simulink model "gm_MATE_HDLsolver_myFirstCircuit"  (R2024b)
settings: Solver=FixedStepDiscrete  StartTime=0.0  StopTime=0.05  FixedStep=6.02409638554217e-09  MaxStep=100e-6  RelTol=1e-4
PostLoadFcn:
  | Ts=1e-6; nb_sw=3; nb_lc=2;nb_r=1;nb_src=1; nb_out=3; rL=1.2;rC=100;L=1e-3; C=1e-5; LpejoSw=1e-6;h=Ts; MAX_INPUTS=16;
  | MAX_OUTPUTS=16;
  | MAX_SWITCHES=8;
  | MAX_INPUTS=16;
InitFcn:
  | Ts=1e-6; nb_sw=3; nb_lc=2;nb_r=1;nb_src=1; nb_out=3; rL=1.2;rC=100;L=1e-3; C=1e-5; LpejoSw=1e-6;h=Ts; MAX_INPUTS=16;
  | MAX_OUTPUTS=16;
  | MAX_SWITCHES=8;
  | MAX_INPUTS=16;
undefined symbols (not defined in the file or in its folder): MATE_SOC
libraries: fl_lib x31, nesl_utility x13, hdlmdlgenlib x10, simetranss x5, simulink x4, hdlsllib x3, ee_lib x2, eeGeneralControl x1
(part 7 of 8)

== system gm_MATE_HDLsolver_myFirstCircuit/ForFPGA/mul_Dot Product5_dotp_11 ==
  In1 : Inport
  In2 : Inport  Port=2
  mul_Dot Product5_dotp_11 : Product  Inputs=**  OutDataTypeStr=single  SampleTime=6.02409638554217e-09
  mul_Dot Product5_dotp_11_pd1 : Delay  DelayLength=6
  Out1 : Outport
  wires:
  In1/1 -> mul_Dot Product5_dotp_11/1
  In2/1 -> mul_Dot Product5_dotp_11/2
  mul_Dot Product5_dotp_11/1 -> mul_Dot Product5_dotp_11_pd1/1
  mul_Dot Product5_dotp_11_pd1/1 -> Out1/1

== system gm_MATE_HDLsolver_myFirstCircuit/ForFPGA/mul_Dot Product5_dotp_12 ==
  In1 : Inport
  In2 : Inport  Port=2
  mul_Dot Product5_dotp_12 : Product  Inputs=**  OutDataTypeStr=single  SampleTime=6.02409638554217e-09
  mul_Dot Product5_dotp_12_pd1 : Delay  DelayLength=6
  Out1 : Outport
  wires:
  In1/1 -> mul_Dot Product5_dotp_12/1
  In2/1 -> mul_Dot Product5_dotp_12/2
  mul_Dot Product5_dotp_12/1 -> mul_Dot Product5_dotp_12_pd1/1
  mul_Dot Product5_dotp_12_pd1/1 -> Out1/1

== system gm_MATE_HDLsolver_myFirstCircuit/ForFPGA/mul_Dot Product5_dotp_13 ==
  In1 : Inport
  In2 : Inport  Port=2
  mul_Dot Product5_dotp_13 : Product  Inputs=**  OutDataTypeStr=single  SampleTime=6.02409638554217e-09
  mul_Dot Product5_dotp_13_pd1 : Delay  DelayLength=6
  Out1 : Outport
  wires:
  In1/1 -> mul_Dot Product5_dotp_13/1
  In2/1 -> mul_Dot Product5_dotp_13/2
  mul_Dot Product5_dotp_13/1 -> mul_Dot Product5_dotp_13_pd1/1
  mul_Dot Product5_dotp_13_pd1/1 -> Out1/1

== system gm_MATE_HDLsolver_myFirstCircuit/ForFPGA/mul_Dot Product5_dotp_14 ==
  In1 : Inport
  In2 : Inport  Port=2
  mul_Dot Product5_dotp_14 : Product  Inputs=**  OutDataTypeStr=single  SampleTime=6.02409638554217e-09
  mul_Dot Product5_dotp_14_pd1 : Delay  DelayLength=6
  Out1 : Outport
  wires:
  In1/1 -> mul_Dot Product5_dotp_14/1
  In2/1 -> mul_Dot Product5_dotp_14/2
  mul_Dot Product5_dotp_14/1 -> mul_Dot Product5_dotp_14_pd1/1
  mul_Dot Product5_dotp_14_pd1/1 -> Out1/1

== system gm_MATE_HDLsolver_myFirstCircuit/ForFPGA/mul_Dot Product5_dotp_15 ==
  In1 : Inport
  In2 : Inport  Port=2
  mul_Dot Product5_dotp_15 : Product  Inputs=**  OutDataTypeStr=single  SampleTime=6.02409638554217e-09
  mul_Dot Product5_dotp_15_pd1 : Delay  DelayLength=6
  Out1 : Outport
  wires:
  In1/1 -> mul_Dot Product5_dotp_15/1
  In2/1 -> mul_Dot Product5_dotp_15/2
  mul_Dot Product5_dotp_15/1 -> mul_Dot Product5_dotp_15_pd1/1
  mul_Dot Product5_dotp_15_pd1/1 -> Out1/1

== system gm_MATE_HDLsolver_myFirstCircuit/ForFPGA/mul_Dot Product5_dotp_2 ==
  In1 : Inport
  In2 : Inport  Port=2
  mul_Dot Product5_dotp_2 : Product  Inputs=**  OutDataTypeStr=single  SampleTime=6.02409638554217e-09
  mul_Dot Product5_dotp_2_pd1 : Delay  DelayLength=6
  Out1 : Outport
  wires:
  In1/1 -> mul_Dot Product5_dotp_2/1
  In2/1 -> mul_Dot Product5_dotp_2/2
  mul_Dot Product5_dotp_2/1 -> mul_Dot Product5_dotp_2_pd1/1
  mul_Dot Product5_dotp_2_pd1/1 -> Out1/1

== system gm_MATE_HDLsolver_myFirstCircuit/ForFPGA/mul_Dot Product5_dotp_3 ==
  In1 : Inport
  In2 : Inport  Port=2
  mul_Dot Product5_dotp_3 : Product  Inputs=**  OutDataTypeStr=single  SampleTime=6.02409638554217e-09
  mul_Dot Product5_dotp_3_pd1 : Delay  DelayLength=6
  Out1 : Outport
  wires:
  In1/1 -> mul_Dot Product5_dotp_3/1
  In2/1 -> mul_Dot Product5_dotp_3/2
  mul_Dot Product5_dotp_3/1 -> mul_Dot Product5_dotp_3_pd1/1
  mul_Dot Product5_dotp_3_pd1/1 -> Out1/1

== system gm_MATE_HDLsolver_myFirstCircuit/ForFPGA/mul_Dot Product5_dotp_4 ==
  In1 : Inport
  In2 : Inport  Port=2
  mul_Dot Product5_dotp_4 : Product  Inputs=**  OutDataTypeStr=single  SampleTime=6.02409638554217e-09
  mul_Dot Product5_dotp_4_pd1 : Delay  DelayLength=6
  Out1 : Outport
  wires:
  In1/1 -> mul_Dot Product5_dotp_4/1
  In2/1 -> mul_Dot Product5_dotp_4/2
  mul_Dot Product5_dotp_4/1 -> mul_Dot Product5_dotp_4_pd1/1
  mul_Dot Product5_dotp_4_pd1/1 -> Out1/1

== system gm_MATE_HDLsolver_myFirstCircuit/ForFPGA/mul_Dot Product5_dotp_5 ==
  In1 : Inport
  In2 : Inport  Port=2
  mul_Dot Product5_dotp_5 : Product  Inputs=**  OutDataTypeStr=single  SampleTime=6.02409638554217e-09
  mul_Dot Product5_dotp_5_pd1 : Delay  DelayLength=6
  Out1 : Outport
  wires:
  In1/1 -> mul_Dot Product5_dotp_5/1
  In2/1 -> mul_Dot Product5_dotp_5/2
  mul_Dot Product5_dotp_5/1 -> mul_Dot Product5_dotp_5_pd1/1
  mul_Dot Product5_dotp_5_pd1/1 -> Out1/1

== system gm_MATE_HDLsolver_myFirstCircuit/ForFPGA/mul_Dot Product5_dotp_6 ==
  In1 : Inport
  In2 : Inport  Port=2
  mul_Dot Product5_dotp_6 : Product  Inputs=**  OutDataTypeStr=single  SampleTime=6.02409638554217e-09
  mul_Dot Product5_dotp_6_pd1 : Delay  DelayLength=6
  Out1 : Outport
  wires:
  In1/1 -> mul_Dot Product5_dotp_6/1
  In2/1 -> mul_Dot Product5_dotp_6/2
  mul_Dot Product5_dotp_6/1 -> mul_Dot Product5_dotp_6_pd1/1
  mul_Dot Product5_dotp_6_pd1/1 -> Out1/1

== system gm_MATE_HDLsolver_myFirstCircuit/ForFPGA/mul_Dot Product5_dotp_7 ==
  In1 : Inport
  In2 : Inport  Port=2
  mul_Dot Product5_dotp_7 : Product  Inputs=**  OutDataTypeStr=single  SampleTime=6.02409638554217e-09
  mul_Dot Product5_dotp_7_pd1 : Delay  DelayLength=6
  Out1 : Outport
  wires:
  In1/1 -> mul_Dot Product5_dotp_7/1
  In2/1 -> mul_Dot Product5_dotp_7/2
  mul_Dot Product5_dotp_7/1 -> mul_Dot Product5_dotp_7_pd1/1
  mul_Dot Product5_dotp_7_pd1/1 -> Out1/1

== system gm_MATE_HDLsolver_myFirstCircuit/ForFPGA/mul_Dot Product5_dotp_8 ==
  In1 : Inport
  In2 : Inport  Port=2
  mul_Dot Product5_dotp_8 : Product  Inputs=**  OutDataTypeStr=single  SampleTime=6.02409638554217e-09
  mul_Dot Product5_dotp_8_pd1 : Delay  DelayLength=6
  Out1 : Outport
  wires:
  In1/1 -> mul_Dot Product5_dotp_8/1
  In2/1 -> mul_Dot Product5_dotp_8/2
  mul_Dot Product5_dotp_8/1 -> mul_Dot Product5_dotp_8_pd1/1
  mul_Dot Product5_dotp_8_pd1/1 -> Out1/1

== system gm_MATE_HDLsolver_myFirstCircuit/ForFPGA/mul_Dot Product5_dotp_9 ==
  In1 : Inport
  In2 : Inport  Port=2
  mul_Dot Product5_dotp_9 : Product  Inputs=**  OutDataTypeStr=single  SampleTime=6.02409638554217e-09
  mul_Dot Product5_dotp_9_pd1 : Delay  DelayLength=6
  Out1 : Outport
  wires:
  In1/1 -> mul_Dot Product5_dotp_9/1
  In2/1 -> mul_Dot Product5_dotp_9/2
  mul_Dot Product5_dotp_9/1 -> mul_Dot Product5_dotp_9_pd1/1
  mul_Dot Product5_dotp_9_pd1/1 -> Out1/1

== system gm_MATE_HDLsolver_myFirstCircuit/ForFPGA/mul_Dot Product6_dotp_0 ==
  In1 : Inport
  In2 : Inport  Port=2
  mul_Dot Product6_dotp_0 : Product  Inputs=**  OutDataTypeStr=single  SampleTime=6.02409638554217e-09
  mul_Dot Product6_dotp_0_pd1 : Delay  DelayLength=6
  Out1 : Outport
  wires:
  In1/1 -> mul_Dot Product6_dotp_0/1
  In2/1 -> mul_Dot Product6_dotp_0/2
  mul_Dot Product6_dotp_0/1 -> mul_Dot Product6_dotp_0_pd1/1
  mul_Dot Product6_dotp_0_pd1/1 -> Out1/1

== system gm_MATE_HDLsolver_myFirstCircuit/ForFPGA/mul_Dot Product6_dotp_1 ==
  In1 : Inport
  In2 : Inport  Port=2
  mul_Dot Product6_dotp_1 : Product  Inputs=**  OutDataTypeStr=single  SampleTime=6.02409638554217e-09
  mul_Dot Product6_dotp_1_pd1 : Delay  DelayLength=6
  Out1 : Outport
  wires:
  In1/1 -> mul_Dot Product6_dotp_1/1
  In2/1 -> mul_Dot Product6_dotp_1/2
  mul_Dot Product6_dotp_1/1 -> mul_Dot Product6_dotp_1_pd1/1
  mul_Dot Product6_dotp_1_pd1/1 -> Out1/1

== system gm_MATE_HDLsolver_myFirstCircuit/ForFPGA/mul_Dot Product6_dotp_10 ==
  In1 : Inport
  In2 : Inport  Port=2
  mul_Dot Product6_dotp_10 : Product  Inputs=**  OutDataTypeStr=single  SampleTime=6.02409638554217e-09
  mul_Dot Product6_dotp_10_pd1 : Delay  DelayLength=6
  Out1 : Outport
  wires:
  In1/1 -> mul_Dot Product6_dotp_10/1
  In2/1 -> mul_Dot Product6_dotp_10/2
  mul_Dot Product6_dotp_10/1 -> mul_Dot Product6_dotp_10_pd1/1
  mul_Dot Product6_dotp_10_pd1/1 -> Out1/1

== system gm_MATE_HDLsolver_myFirstCircuit/ForFPGA/mul_Dot Product6_dotp_11 ==
  In1 : Inport
  In2 : Inport  Port=2
  mul_Dot Product6_dotp_11 : Product  Inputs=**  OutDataTypeStr=single  SampleTime=6.02409638554217e-09
  mul_Dot Product6_dotp_11_pd1 : Delay  DelayLength=6
  Out1 : Outport
  wires:
  In1/1 -> mul_Dot Product6_dotp_11/1
  In2/1 -> mul_Dot Product6_dotp_11/2
  mul_Dot Product6_dotp_11/1 -> mul_Dot Product6_dotp_11_pd1/1
  mul_Dot Product6_dotp_11_pd1/1 -> Out1/1

== system gm_MATE_HDLsolver_myFirstCircuit/ForFPGA/mul_Dot Product6_dotp_12 ==
  In1 : Inport
  In2 : Inport  Port=2
  mul_Dot Product6_dotp_12 : Product  Inputs=**  OutDataTypeStr=single  SampleTime=6.02409638554217e-09
  mul_Dot Product6_dotp_12_pd1 : Delay  DelayLength=6
  Out1 : Outport
  wires:
  In1/1 -> mul_Dot Product6_dotp_12/1
  In2/1 -> mul_Dot Product6_dotp_12/2
  mul_Dot Product6_dotp_12/1 -> mul_Dot Product6_dotp_12_pd1/1
  mul_Dot Product6_dotp_12_pd1/1 -> Out1/1

== system gm_MATE_HDLsolver_myFirstCircuit/ForFPGA/mul_Dot Product6_dotp_13 ==
  In1 : Inport
  In2 : Inport  Port=2
  mul_Dot Product6_dotp_13 : Product  Inputs=**  OutDataTypeStr=single  SampleTime=6.02409638554217e-09
  mul_Dot Product6_dotp_13_pd1 : Delay  DelayLength=6
  Out1 : Outport
  wires:
  In1/1 -> mul_Dot Product6_dotp_13/1
  In2/1 -> mul_Dot Product6_dotp_13/2
  mul_Dot Product6_dotp_13/1 -> mul_Dot Product6_dotp_13_pd1/1
  mul_Dot Product6_dotp_13_pd1/1 -> Out1/1

== system gm_MATE_HDLsolver_myFirstCircuit/ForFPGA/mul_Dot Product6_dotp_14 ==
  In1 : Inport
  In2 : Inport  Port=2
  mul_Dot Product6_dotp_14 : Product  Inputs=**  OutDataTypeStr=single  SampleTime=6.02409638554217e-09
  mul_Dot Product6_dotp_14_pd1 : Delay  DelayLength=6
  Out1 : Outport
  wires:
  In1/1 -> mul_Dot Product6_dotp_14/1
  In2/1 -> mul_Dot Product6_dotp_14/2
  mul_Dot Product6_dotp_14/1 -> mul_Dot Product6_dotp_14_pd1/1
  mul_Dot Product6_dotp_14_pd1/1 -> Out1/1

== system gm_MATE_HDLsolver_myFirstCircuit/ForFPGA/mul_Dot Product6_dotp_15 ==
  In1 : Inport
  In2 : Inport  Port=2
  mul_Dot Product6_dotp_15 : Product  Inputs=**  OutDataTypeStr=single  SampleTime=6.02409638554217e-09
  mul_Dot Product6_dotp_15_pd1 : Delay  DelayLength=6
  Out1 : Outport
  wires:
  In1/1 -> mul_Dot Product6_dotp_15/1
  In2/1 -> mul_Dot Product6_dotp_15/2
  mul_Dot Product6_dotp_15/1 -> mul_Dot Product6_dotp_15_pd1/1
  mul_Dot Product6_dotp_15_pd1/1 -> Out1/1

== system gm_MATE_HDLsolver_myFirstCircuit/ForFPGA/mul_Dot Product6_dotp_2 ==
  In1 : Inport
  In2 : Inport  Port=2
  mul_Dot Product6_dotp_2 : Product  Inputs=**  OutDataTypeStr=single  SampleTime=6.02409638554217e-09
  mul_Dot Product6_dotp_2_pd1 : Delay  DelayLength=6
  Out1 : Outport
  wires:
  In1/1 -> mul_Dot Product6_dotp_2/1
  In2/1 -> mul_Dot Product6_dotp_2/2
  mul_Dot Product6_dotp_2/1 -> mul_Dot Product6_dotp_2_pd1/1
  mul_Dot Product6_dotp_2_pd1/1 -> Out1/1

== system gm_MATE_HDLsolver_myFirstCircuit/ForFPGA/mul_Dot Product6_dotp_3 ==
  In1 : Inport
  In2 : Inport  Port=2
  mul_Dot Product6_dotp_3 : Product  Inputs=**  OutDataTypeStr=single  SampleTime=6.02409638554217e-09
  mul_Dot Product6_dotp_3_pd1 : Delay  DelayLength=6
  Out1 : Outport
  wires:
  In1/1 -> mul_Dot Product6_dotp_3/1
  In2/1 -> mul_Dot Product6_dotp_3/2
  mul_Dot Product6_dotp_3/1 -> mul_Dot Product6_dotp_3_pd1/1
  mul_Dot Product6_dotp_3_pd1/1 -> Out1/1

== system gm_MATE_HDLsolver_myFirstCircuit/ForFPGA/mul_Dot Product6_dotp_4 ==
  In1 : Inport
  In2 : Inport  Port=2
  mul_Dot Product6_dotp_4 : Product  Inputs=**  OutDataTypeStr=single  SampleTime=6.02409638554217e-09
  mul_Dot Product6_dotp_4_pd1 : Delay  DelayLength=6
  Out1 : Outport
  wires:
  In1/1 -> mul_Dot Product6_dotp_4/1
  In2/1 -> mul_Dot Product6_dotp_4/2
  mul_Dot Product6_dotp_4/1 -> mul_Dot Product6_dotp_4_pd1/1
  mul_Dot Product6_dotp_4_pd1/1 -> Out1/1

== system gm_MATE_HDLsolver_myFirstCircuit/ForFPGA/mul_Dot Product6_dotp_5 ==
  In1 : Inport
  In2 : Inport  Port=2
  mul_Dot Product6_dotp_5 : Product  Inputs=**  OutDataTypeStr=single  SampleTime=6.02409638554217e-09
  mul_Dot Product6_dotp_5_pd1 : Delay  DelayLength=6
  Out1 : Outport
  wires:
  In1/1 -> mul_Dot Product6_dotp_5/1
  In2/1 -> mul_Dot Product6_dotp_5/2
  mul_Dot Product6_dotp_5/1 -> mul_Dot Product6_dotp_5_pd1/1
  mul_Dot Product6_dotp_5_pd1/1 -> Out1/1

== system gm_MATE_HDLsolver_myFirstCircuit/ForFPGA/mul_Dot Product6_dotp_6 ==
  In1 : Inport
  In2 : Inport  Port=2
  mul_Dot Product6_dotp_6 : Product  Inputs=**  OutDataTypeStr=single  SampleTime=6.02409638554217e-09
  mul_Dot Product6_dotp_6_pd1 : Delay  DelayLength=6
  Out1 : Outport
  wires:
  In1/1 -> mul_Dot Product6_dotp_6/1
  In2/1 -> mul_Dot Product6_dotp_6/2
  mul_Dot Product6_dotp_6/1 -> mul_Dot Product6_dotp_6_pd1/1
  mul_Dot Product6_dotp_6_pd1/1 -> Out1/1

== system gm_MATE_HDLsolver_myFirstCircuit/ForFPGA/mul_Dot Product6_dotp_7 ==
  In1 : Inport
  In2 : Inport  Port=2
  mul_Dot Product6_dotp_7 : Product  Inputs=**  OutDataTypeStr=single  SampleTime=6.02409638554217e-09
  mul_Dot Product6_dotp_7_pd1 : Delay  DelayLength=6
  Out1 : Outport
  wires:
  In1/1 -> mul_Dot Product6_dotp_7/1
  In2/1 -> mul_Dot Product6_dotp_7/2
  mul_Dot Product6_dotp_7/1 -> mul_Dot Product6_dotp_7_pd1/1
  mul_Dot Product6_dotp_7_pd1/1 -> Out1/1

== system gm_MATE_HDLsolver_myFirstCircuit/ForFPGA/mul_Dot Product6_dotp_8 ==
  In1 : Inport
  In2 : Inport  Port=2
  mul_Dot Product6_dotp_8 : Product  Inputs=**  OutDataTypeStr=single  SampleTime=6.02409638554217e-09
  mul_Dot Product6_dotp_8_pd1 : Delay  DelayLength=6
  Out1 : Outport
  wires:
  In1/1 -> mul_Dot Product6_dotp_8/1
  In2/1 -> mul_Dot Product6_dotp_8/2
  mul_Dot Product6_dotp_8/1 -> mul_Dot Product6_dotp_8_pd1/1
  mul_Dot Product6_dotp_8_pd1/1 -> Out1/1

== system gm_MATE_HDLsolver_myFirstCircuit/ForFPGA/mul_Dot Product6_dotp_9 ==
  In1 : Inport
  In2 : Inport  Port=2
  mul_Dot Product6_dotp_9 : Product  Inputs=**  OutDataTypeStr=single  SampleTime=6.02409638554217e-09
  mul_Dot Product6_dotp_9_pd1 : Delay  DelayLength=6
  Out1 : Outport
  wires:
  In1/1 -> mul_Dot Product6_dotp_9/1
  In2/1 -> mul_Dot Product6_dotp_9/2
  mul_Dot Product6_dotp_9/1 -> mul_Dot Product6_dotp_9_pd1/1
  mul_Dot Product6_dotp_9_pd1/1 -> Out1/1

== system gm_MATE_HDLsolver_myFirstCircuit/ForFPGA/mul_Dot Product7_dotp_0 ==
  In1 : Inport
  In2 : Inport  Port=2
  mul_Dot Product7_dotp_0 : Product  Inputs=**  OutDataTypeStr=single  SampleTime=6.02409638554217e-09
  mul_Dot Product7_dotp_0_pd1 : Delay  DelayLength=6
  Out1 : Outport
  wires:
  In1/1 -> mul_Dot Product7_dotp_0/1
  In2/1 -> mul_Dot Product7_dotp_0/2
  mul_Dot Product7_dotp_0/1 -> mul_Dot Product7_dotp_0_pd1/1
  mul_Dot Product7_dotp_0_pd1/1 -> Out1/1

== system gm_MATE_HDLsolver_myFirstCircuit/ForFPGA/mul_Dot Product7_dotp_1 ==
  In1 : Inport
  In2 : Inport  Port=2
  mul_Dot Product7_dotp_1 : Product  Inputs=**  OutDataTypeStr=single  SampleTime=6.02409638554217e-09
  mul_Dot Product7_dotp_1_pd1 : Delay  DelayLength=6
  Out1 : Outport
  wires:
  In1/1 -> mul_Dot Product7_dotp_1/1
  In2/1 -> mul_Dot Product7_dotp_1/2
  mul_Dot Product7_dotp_1/1 -> mul_Dot Product7_dotp_1_pd1/1
  mul_Dot Product7_dotp_1_pd1/1 -> Out1/1

== system gm_MATE_HDLsolver_myFirstCircuit/ForFPGA/mul_Dot Product7_dotp_10 ==
  In1 : Inport
  In2 : Inport  Port=2
  mul_Dot Product7_dotp_10 : Product  Inputs=**  OutDataTypeStr=single  SampleTime=6.02409638554217e-09
  mul_Dot Product7_dotp_10_pd1 : Delay  DelayLength=6
  Out1 : Outport
  wires:
  In1/1 -> mul_Dot Product7_dotp_10/1
  In2/1 -> mul_Dot Product7_dotp_10/2
  mul_Dot Product7_dotp_10/1 -> mul_Dot Product7_dotp_10_pd1/1
  mul_Dot Product7_dotp_10_pd1/1 -> Out1/1

== system gm_MATE_HDLsolver_myFirstCircuit/ForFPGA/mul_Dot Product7_dotp_11 ==
  In1 : Inport
  In2 : Inport  Port=2
  mul_Dot Product7_dotp_11 : Product  Inputs=**  OutDataTypeStr=single  SampleTime=6.02409638554217e-09
  mul_Dot Product7_dotp_11_pd1 : Delay  DelayLength=6
  Out1 : Outport
  wires:
  In1/1 -> mul_Dot Product7_dotp_11/1
  In2/1 -> mul_Dot Product7_dotp_11/2
  mul_Dot Product7_dotp_11/1 -> mul_Dot Product7_dotp_11_pd1/1
  mul_Dot Product7_dotp_11_pd1/1 -> Out1/1

== system gm_MATE_HDLsolver_myFirstCircuit/ForFPGA/mul_Dot Product7_dotp_12 ==
  In1 : Inport
  In2 : Inport  Port=2
  mul_Dot Product7_dotp_12 : Product  Inputs=**  OutDataTypeStr=single  SampleTime=6.02409638554217e-09
  mul_Dot Product7_dotp_12_pd1 : Delay  DelayLength=6
  Out1 : Outport
  wires:
  In1/1 -> mul_Dot Product7_dotp_12/1
  In2/1 -> mul_Dot Product7_dotp_12/2
  mul_Dot Product7_dotp_12/1 -> mul_Dot Product7_dotp_12_pd1/1
  mul_Dot Product7_dotp_12_pd1/1 -> Out1/1

== system gm_MATE_HDLsolver_myFirstCircuit/ForFPGA/mul_Dot Product7_dotp_13 ==
  In1 : Inport
  In2 : Inport  Port=2
  mul_Dot Product7_dotp_13 : Product  Inputs=**  OutDataTypeStr=single  SampleTime=6.02409638554217e-09
  mul_Dot Product7_dotp_13_pd1 : Delay  DelayLength=6
  Out1 : Outport
  wires:
  In1/1 -> mul_Dot Product7_dotp_13/1
  In2/1 -> mul_Dot Product7_dotp_13/2
  mul_Dot Product7_dotp_13/1 -> mul_Dot Product7_dotp_13_pd1/1
  mul_Dot Product7_dotp_13_pd1/1 -> Out1/1

== system gm_MATE_HDLsolver_myFirstCircuit/ForFPGA/mul_Dot Product7_dotp_14 ==
  In1 : Inport
  In2 : Inport  Port=2
  mul_Dot Product7_dotp_14 : Product  Inputs=**  OutDataTypeStr=single  SampleTime=6.02409638554217e-09
  mul_Dot Product7_dotp_14_pd1 : Delay  DelayLength=6
  Out1 : Outport
  wires:
  In1/1 -> mul_Dot Product7_dotp_14/1
  In2/1 -> mul_Dot Product7_dotp_14/2
  mul_Dot Product7_dotp_14/1 -> mul_Dot Product7_dotp_14_pd1/1
  mul_Dot Product7_dotp_14_pd1/1 -> Out1/1

== system gm_MATE_HDLsolver_myFirstCircuit/ForFPGA/mul_Dot Product7_dotp_15 ==
  In1 : Inport
  In2 : Inport  Port=2
  mul_Dot Product7_dotp_15 : Product  Inputs=**  OutDataTypeStr=single  SampleTime=6.02409638554217e-09
  mul_Dot Product7_dotp_15_pd1 : Delay  DelayLength=6
  Out1 : Outport
  wires:
  In1/1 -> mul_Dot Product7_dotp_15/1
  In2/1 -> mul_Dot Product7_dotp_15/2
  mul_Dot Product7_dotp_15/1 -> mul_Dot Product7_dotp_15_pd1/1
  mul_Dot Product7_dotp_15_pd1/1 -> Out1/1

== system gm_MATE_HDLsolver_myFirstCircuit/ForFPGA/mul_Dot Product7_dotp_2 ==
  In1 : Inport
  In2 : Inport  Port=2
  mul_Dot Product7_dotp_2 : Product  Inputs=**  OutDataTypeStr=single  SampleTime=6.02409638554217e-09
  mul_Dot Product7_dotp_2_pd1 : Delay  DelayLength=6
  Out1 : Outport
  wires:
  In1/1 -> mul_Dot Product7_dotp_2/1
  In2/1 -> mul_Dot Product7_dotp_2/2
  mul_Dot Product7_dotp_2/1 -> mul_Dot Product7_dotp_2_pd1/1
  mul_Dot Product7_dotp_2_pd1/1 -> Out1/1

== system gm_MATE_HDLsolver_myFirstCircuit/ForFPGA/mul_Dot Product7_dotp_3 ==
  In1 : Inport
  In2 : Inport  Port=2
  mul_Dot Product7_dotp_3 : Product  Inputs=**  OutDataTypeStr=single  SampleTime=6.02409638554217e-09
  mul_Dot Product7_dotp_3_pd1 : Delay  DelayLength=6
  Out1 : Outport
  wires:
  In1/1 -> mul_Dot Product7_dotp_3/1
  In2/1 -> mul_Dot Product7_dotp_3/2
  mul_Dot Product7_dotp_3/1 -> mul_Dot Product7_dotp_3_pd1/1
  mul_Dot Product7_dotp_3_pd1/1 -> Out1/1

== system gm_MATE_HDLsolver_myFirstCircuit/ForFPGA/mul_Dot Product7_dotp_4 ==
  In1 : Inport
  In2 : Inport  Port=2
  mul_Dot Product7_dotp_4 : Product  Inputs=**  OutDataTypeStr=single  SampleTime=6.02409638554217e-09
  mul_Dot Product7_dotp_4_pd1 : Delay  DelayLength=6
  Out1 : Outport
  wires:
  In1/1 -> mul_Dot Product7_dotp_4/1
  In2/1 -> mul_Dot Product7_dotp_4/2
  mul_Dot Product7_dotp_4/1 -> mul_Dot Product7_dotp_4_pd1/1
  mul_Dot Product7_dotp_4_pd1/1 -> Out1/1

== system gm_MATE_HDLsolver_myFirstCircuit/ForFPGA/mul_Dot Product7_dotp_5 ==
  In1 : Inport
  In2 : Inport  Port=2
  mul_Dot Product7_dotp_5 : Product  Inputs=**  OutDataTypeStr=single  SampleTime=6.02409638554217e-09
  mul_Dot Product7_dotp_5_pd1 : Delay  DelayLength=6
  Out1 : Outport
  wires:
  In1/1 -> mul_Dot Product7_dotp_5/1
  In2/1 -> mul_Dot Product7_dotp_5/2
  mul_Dot Product7_dotp_5/1 -> mul_Dot Product7_dotp_5_pd1/1
  mul_Dot Product7_dotp_5_pd1/1 -> Out1/1

== system gm_MATE_HDLsolver_myFirstCircuit/ForFPGA/mul_Dot Product7_dotp_6 ==
  In1 : Inport
  In2 : Inport  Port=2
  mul_Dot Product7_dotp_6 : Product  Inputs=**  OutDataTypeStr=single  SampleTime=6.02409638554217e-09
  mul_Dot Product7_dotp_6_pd1 : Delay  DelayLength=6
  Out1 : Outport
  wires:
  In1/1 -> mul_Dot Product7_dotp_6/1
  In2/1 -> mul_Dot Product7_dotp_6/2
  mul_Dot Product7_dotp_6/1 -> mul_Dot Product7_dotp_6_pd1/1
  mul_Dot Product7_dotp_6_pd1/1 -> Out1/1

== system gm_MATE_HDLsolver_myFirstCircuit/ForFPGA/mul_Dot Product7_dotp_7 ==
  In1 : Inport
  In2 : Inport  Port=2
  mul_Dot Product7_dotp_7 : Product  Inputs=**  OutDataTypeStr=single  SampleTime=6.02409638554217e-09
  mul_Dot Product7_dotp_7_pd1 : Delay  DelayLength=6
  Out1 : Outport
  wires:
  In1/1 -> mul_Dot Product7_dotp_7/1
  In2/1 -> mul_Dot Product7_dotp_7/2
  mul_Dot Product7_dotp_7/1 -> mul_Dot Product7_dotp_7_pd1/1
  mul_Dot Product7_dotp_7_pd1/1 -> Out1/1

== system gm_MATE_HDLsolver_myFirstCircuit/ForFPGA/mul_Dot Product7_dotp_8 ==
  In1 : Inport
  In2 : Inport  Port=2
  mul_Dot Product7_dotp_8 : Product  Inputs=**  OutDataTypeStr=single  SampleTime=6.02409638554217e-09
  mul_Dot Product7_dotp_8_pd1 : Delay  DelayLength=6
  Out1 : Outport
  wires:
  In1/1 -> mul_Dot Product7_dotp_8/1
  In2/1 -> mul_Dot Product7_dotp_8/2
  mul_Dot Product7_dotp_8/1 -> mul_Dot Product7_dotp_8_pd1/1
  mul_Dot Product7_dotp_8_pd1/1 -> Out1/1

== system gm_MATE_HDLsolver_myFirstCircuit/ForFPGA/mul_Dot Product7_dotp_9 ==
  In1 : Inport
  In2 : Inport  Port=2
  mul_Dot Product7_dotp_9 : Product  Inputs=**  OutDataTypeStr=single  SampleTime=6.02409638554217e-09
  mul_Dot Product7_dotp_9_pd1 : Delay  DelayLength=6
  Out1 : Outport
  wires:
  In1/1 -> mul_Dot Product7_dotp_9/1
  In2/1 -> mul_Dot Product7_dotp_9/2
  mul_Dot Product7_dotp_9/1 -> mul_Dot Product7_dotp_9_pd1/1
  mul_Dot Product7_dotp_9_pd1/1 -> Out1/1

== system gm_MATE_HDLsolver_myFirstCircuit/ForFPGA/mul_Dot Product8_dotp_0 ==
  In1 : Inport
  In2 : Inport  Port=2
  mul_Dot Product8_dotp_0 : Product  Inputs=**  OutDataTypeStr=single  SampleTime=6.02409638554217e-09
  mul_Dot Product8_dotp_0_pd1 : Delay  DelayLength=6
  Out1 : Outport
  wires:
  In1/1 -> mul_Dot Product8_dotp_0/1
  In2/1 -> mul_Dot Product8_dotp_0/2
  mul_Dot Product8_dotp_0/1 -> mul_Dot Product8_dotp_0_pd1/1
  mul_Dot Product8_dotp_0_pd1/1 -> Out1/1

== system gm_MATE_HDLsolver_myFirstCircuit/ForFPGA/mul_Dot Product8_dotp_1 ==
  In1 : Inport
  In2 : Inport  Port=2
  mul_Dot Product8_dotp_1 : Product  Inputs=**  OutDataTypeStr=single  SampleTime=6.02409638554217e-09
  mul_Dot Product8_dotp_1_pd1 : Delay  DelayLength=6
  Out1 : Outport
  wires:
  In1/1 -> mul_Dot Product8_dotp_1/1
  In2/1 -> mul_Dot Product8_dotp_1/2
  mul_Dot Product8_dotp_1/1 -> mul_Dot Product8_dotp_1_pd1/1
  mul_Dot Product8_dotp_1_pd1/1 -> Out1/1

== system gm_MATE_HDLsolver_myFirstCircuit/ForFPGA/mul_Dot Product8_dotp_10 ==
  In1 : Inport
  In2 : Inport  Port=2
  mul_Dot Product8_dotp_10 : Product  Inputs=**  OutDataTypeStr=single  SampleTime=6.02409638554217e-09
  mul_Dot Product8_dotp_10_pd1 : Delay  DelayLength=6
  Out1 : Outport
  wires:
  In1/1 -> mul_Dot Product8_dotp_10/1
  In2/1 -> mul_Dot Product8_dotp_10/2
  mul_Dot Product8_dotp_10/1 -> mul_Dot Product8_dotp_10_pd1/1
  mul_Dot Product8_dotp_10_pd1/1 -> Out1/1

== system gm_MATE_HDLsolver_myFirstCircuit/ForFPGA/mul_Dot Product8_dotp_11 ==
  In1 : Inport
  In2 : Inport  Port=2
  mul_Dot Product8_dotp_11 : Product  Inputs=**  OutDataTypeStr=single  SampleTime=6.02409638554217e-09
  mul_Dot Product8_dotp_11_pd1 : Delay  DelayLength=6
  Out1 : Outport
  wires:
  In1/1 -> mul_Dot Product8_dotp_11/1
  In2/1 -> mul_Dot Product8_dotp_11/2
  mul_Dot Product8_dotp_11/1 -> mul_Dot Product8_dotp_11_pd1/1
  mul_Dot Product8_dotp_11_pd1/1 -> Out1/1

== system gm_MATE_HDLsolver_myFirstCircuit/ForFPGA/mul_Dot Product8_dotp_12 ==
  In1 : Inport
  In2 : Inport  Port=2
  mul_Dot Product8_dotp_12 : Product  Inputs=**  OutDataTypeStr=single  SampleTime=6.02409638554217e-09
  mul_Dot Product8_dotp_12_pd1 : Delay  DelayLength=6
  Out1 : Outport
  wires:
  In1/1 -> mul_Dot Product8_dotp_12/1
  In2/1 -> mul_Dot Product8_dotp_12/2
  mul_Dot Product8_dotp_12/1 -> mul_Dot Product8_dotp_12_pd1/1
  mul_Dot Product8_dotp_12_pd1/1 -> Out1/1

== system gm_MATE_HDLsolver_myFirstCircuit/ForFPGA/mul_Dot Product8_dotp_13 ==
  In1 : Inport
  In2 : Inport  Port=2
  mul_Dot Product8_dotp_13 : Product  Inputs=**  OutDataTypeStr=single  SampleTime=6.02409638554217e-09
  mul_Dot Product8_dotp_13_pd1 : Delay  DelayLength=6
  Out1 : Outport
  wires:
  In1/1 -> mul_Dot Product8_dotp_13/1
  In2/1 -> mul_Dot Product8_dotp_13/2
  mul_Dot Product8_dotp_13/1 -> mul_Dot Product8_dotp_13_pd1/1
  mul_Dot Product8_dotp_13_pd1/1 -> Out1/1

== system gm_MATE_HDLsolver_myFirstCircuit/ForFPGA/mul_Dot Product8_dotp_14 ==
  In1 : Inport
  In2 : Inport  Port=2
  mul_Dot Product8_dotp_14 : Product  Inputs=**  OutDataTypeStr=single  SampleTime=6.02409638554217e-09
  mul_Dot Product8_dotp_14_pd1 : Delay  DelayLength=6
  Out1 : Outport
  wires:
  In1/1 -> mul_Dot Product8_dotp_14/1
  In2/1 -> mul_Dot Product8_dotp_14/2
  mul_Dot Product8_dotp_14/1 -> mul_Dot Product8_dotp_14_pd1/1
  mul_Dot Product8_dotp_14_pd1/1 -> Out1/1

== system gm_MATE_HDLsolver_myFirstCircuit/ForFPGA/mul_Dot Product8_dotp_15 ==
  In1 : Inport
  In2 : Inport  Port=2
  mul_Dot Product8_dotp_15 : Product  Inputs=**  OutDataTypeStr=single  SampleTime=6.02409638554217e-09
  mul_Dot Product8_dotp_15_pd1 : Delay  DelayLength=6
  Out1 : Outport
  wires:
  In1/1 -> mul_Dot Product8_dotp_15/1
  In2/1 -> mul_Dot Product8_dotp_15/2
  mul_Dot Product8_dotp_15/1 -> mul_Dot Product8_dotp_15_pd1/1
  mul_Dot Product8_dotp_15_pd1/1 -> Out1/1

== system gm_MATE_HDLsolver_myFirstCircuit/ForFPGA/mul_Dot Product8_dotp_2 ==
  In1 : Inport
  In2 : Inport  Port=2
  mul_Dot Product8_dotp_2 : Product  Inputs=**  OutDataTypeStr=single  SampleTime=6.02409638554217e-09
  mul_Dot Product8_dotp_2_pd1 : Delay  DelayLength=6
  Out1 : Outport
  wires:
  In1/1 -> mul_Dot Product8_dotp_2/1
  In2/1 -> mul_Dot Product8_dotp_2/2
  mul_Dot Product8_dotp_2/1 -> mul_Dot Product8_dotp_2_pd1/1
  mul_Dot Product8_dotp_2_pd1/1 -> Out1/1

== system gm_MATE_HDLsolver_myFirstCircuit/ForFPGA/mul_Dot Product8_dotp_3 ==
  In1 : Inport
  In2 : Inport  Port=2
  mul_Dot Product8_dotp_3 : Product  Inputs=**  OutDataTypeStr=single  SampleTime=6.02409638554217e-09
  mul_Dot Product8_dotp_3_pd1 : Delay  DelayLength=6
  Out1 : Outport
  wires:
  In1/1 -> mul_Dot Product8_dotp_3/1
  In2/1 -> mul_Dot Product8_dotp_3/2
  mul_Dot Product8_dotp_3/1 -> mul_Dot Product8_dotp_3_pd1/1
  mul_Dot Product8_dotp_3_pd1/1 -> Out1/1

== system gm_MATE_HDLsolver_myFirstCircuit/ForFPGA/mul_Dot Product8_dotp_4 ==
  In1 : Inport
  In2 : Inport  Port=2
  mul_Dot Product8_dotp_4 : Product  Inputs=**  OutDataTypeStr=single  SampleTime=6.02409638554217e-09
  mul_Dot Product8_dotp_4_pd1 : Delay  DelayLength=6
  Out1 : Outport
  wires:
  In1/1 -> mul_Dot Product8_dotp_4/1
  In2/1 -> mul_Dot Product8_dotp_4/2
  mul_Dot Product8_dotp_4/1 -> mul_Dot Product8_dotp_4_pd1/1
  mul_Dot Product8_dotp_4_pd1/1 -> Out1/1

== system gm_MATE_HDLsolver_myFirstCircuit/ForFPGA/mul_Dot Product8_dotp_5 ==
  In1 : Inport
  In2 : Inport  Port=2
  mul_Dot Product8_dotp_5 : Product  Inputs=**  OutDataTypeStr=single  SampleTime=6.02409638554217e-09
  mul_Dot Product8_dotp_5_pd1 : Delay  DelayLength=6
  Out1 : Outport
  wires:
  In1/1 -> mul_Dot Product8_dotp_5/1
  In2/1 -> mul_Dot Product8_dotp_5/2
  mul_Dot Product8_dotp_5/1 -> mul_Dot Product8_dotp_5_pd1/1
  mul_Dot Product8_dotp_5_pd1/1 -> Out1/1

== system gm_MATE_HDLsolver_myFirstCircuit/ForFPGA/mul_Dot Product8_dotp_6 ==
  In1 : Inport
  In2 : Inport  Port=2
  mul_Dot Product8_dotp_6 : Product  Inputs=**  OutDataTypeStr=single  SampleTime=6.02409638554217e-09
  mul_Dot Product8_dotp_6_pd1 : Delay  DelayLength=6
  Out1 : Outport
  wires:
  In1/1 -> mul_Dot Product8_dotp_6/1
  In2/1 -> mul_Dot Product8_dotp_6/2
  mul_Dot Product8_dotp_6/1 -> mul_Dot Product8_dotp_6_pd1/1
  mul_Dot Product8_dotp_6_pd1/1 -> Out1/1

== system gm_MATE_HDLsolver_myFirstCircuit/ForFPGA/mul_Dot Product8_dotp_7 ==
  In1 : Inport
  In2 : Inport  Port=2
  mul_Dot Product8_dotp_7 : Product  Inputs=**  OutDataTypeStr=single  SampleTime=6.02409638554217e-09
  mul_Dot Product8_dotp_7_pd1 : Delay  DelayLength=6
  Out1 : Outport
  wires:
  In1/1 -> mul_Dot Product8_dotp_7/1
  In2/1 -> mul_Dot Product8_dotp_7/2
  mul_Dot Product8_dotp_7/1 -> mul_Dot Product8_dotp_7_pd1/1
  mul_Dot Product8_dotp_7_pd1/1 -> Out1/1

== system gm_MATE_HDLsolver_myFirstCircuit/ForFPGA/mul_Dot Product8_dotp_8 ==
  In1 : Inport
  In2 : Inport  Port=2
  mul_Dot Product8_dotp_8 : Product  Inputs=**  OutDataTypeStr=single  SampleTime=6.02409638554217e-09
  mul_Dot Product8_dotp_8_pd1 : Delay  DelayLength=6
  Out1 : Outport
  wires:
  In1/1 -> mul_Dot Product8_dotp_8/1
  In2/1 -> mul_Dot Product8_dotp_8/2
  mul_Dot Product8_dotp_8/1 -> mul_Dot Product8_dotp_8_pd1/1
  mul_Dot Product8_dotp_8_pd1/1 -> Out1/1

== system gm_MATE_HDLsolver_myFirstCircuit/ForFPGA/mul_Dot Product8_dotp_9 ==
  In1 : Inport
  In2 : Inport  Port=2
  mul_Dot Product8_dotp_9 : Product  Inputs=**  OutDataTypeStr=single  SampleTime=6.02409638554217e-09
  mul_Dot Product8_dotp_9_pd1 : Delay  DelayLength=6
  Out1 : Outport
  wires:
  In1/1 -> mul_Dot Product8_dotp_9/1
  In2/1 -> mul_Dot Product8_dotp_9/2
  mul_Dot Product8_dotp_9/1 -> mul_Dot Product8_dotp_9_pd1/1
  mul_Dot Product8_dotp_9_pd1/1 -> Out1/1

== system gm_MATE_HDLsolver_myFirstCircuit/ForFPGA/mul_Dot Product9_dotp_0 ==
  In1 : Inport
  In2 : Inport  Port=2
  mul_Dot Product9_dotp_0 : Product  Inputs=**  OutDataTypeStr=single  SampleTime=6.02409638554217e-09
  mul_Dot Product9_dotp_0_pd1 : Delay  DelayLength=6
  Out1 : Outport
  wires:
  In1/1 -> mul_Dot Product9_dotp_0/1
  In2/1 -> mul_Dot Product9_dotp_0/2
  mul_Dot Product9_dotp_0/1 -> mul_Dot Product9_dotp_0_pd1/1
  mul_Dot Product9_dotp_0_pd1/1 -> Out1/1

== system gm_MATE_HDLsolver_myFirstCircuit/ForFPGA/mul_Dot Product9_dotp_1 ==
  In1 : Inport
  In2 : Inport  Port=2
  mul_Dot Product9_dotp_1 : Product  Inputs=**  OutDataTypeStr=single  SampleTime=6.02409638554217e-09
  mul_Dot Product9_dotp_1_pd1 : Delay  DelayLength=6
  Out1 : Outport
  wires:
  In1/1 -> mul_Dot Product9_dotp_1/1
  In2/1 -> mul_Dot Product9_dotp_1/2
  mul_Dot Product9_dotp_1/1 -> mul_Dot Product9_dotp_1_pd1/1
  mul_Dot Product9_dotp_1_pd1/1 -> Out1/1

== system gm_MATE_HDLsolver_myFirstCircuit/ForFPGA/mul_Dot Product9_dotp_10 ==
  In1 : Inport
  In2 : Inport  Port=2
  mul_Dot Product9_dotp_10 : Product  Inputs=**  OutDataTypeStr=single  SampleTime=6.02409638554217e-09
  mul_Dot Product9_dotp_10_pd1 : Delay  DelayLength=6
  Out1 : Outport
  wires:
  In1/1 -> mul_Dot Product9_dotp_10/1
  In2/1 -> mul_Dot Product9_dotp_10/2
  mul_Dot Product9_dotp_10/1 -> mul_Dot Product9_dotp_10_pd1/1
  mul_Dot Product9_dotp_10_pd1/1 -> Out1/1

== system gm_MATE_HDLsolver_myFirstCircuit/ForFPGA/mul_Dot Product9_dotp_11 ==
  In1 : Inport
  In2 : Inport  Port=2
  mul_Dot Product9_dotp_11 : Product  Inputs=**  OutDataTypeStr=single  SampleTime=6.02409638554217e-09
  mul_Dot Product9_dotp_11_pd1 : Delay  DelayLength=6
  Out1 : Outport
  wires:
  In1/1 -> mul_Dot Product9_dotp_11/1
  In2/1 -> mul_Dot Product9_dotp_11/2
  mul_Dot Product9_dotp_11/1 -> mul_Dot Product9_dotp_11_pd1/1
  mul_Dot Product9_dotp_11_pd1/1 -> Out1/1

== system gm_MATE_HDLsolver_myFirstCircuit/ForFPGA/mul_Dot Product9_dotp_12 ==
  In1 : Inport
  In2 : Inport  Port=2
  mul_Dot Product9_dotp_12 : Product  Inputs=**  OutDataTypeStr=single  SampleTime=6.02409638554217e-09
  mul_Dot Product9_dotp_12_pd1 : Delay  DelayLength=6
  Out1 : Outport
  wires:
  In1/1 -> mul_Dot Product9_dotp_12/1
  In2/1 -> mul_Dot Product9_dotp_12/2
  mul_Dot Product9_dotp_12/1 -> mul_Dot Product9_dotp_12_pd1/1
  mul_Dot Product9_dotp_12_pd1/1 -> Out1/1

== system gm_MATE_HDLsolver_myFirstCircuit/ForFPGA/mul_Dot Product9_dotp_13 ==
  In1 : Inport
  In2 : Inport  Port=2
  mul_Dot Product9_dotp_13 : Product  Inputs=**  OutDataTypeStr=single  SampleTime=6.02409638554217e-09
  mul_Dot Product9_dotp_13_pd1 : Delay  DelayLength=6
  Out1 : Outport
  wires:
  In1/1 -> mul_Dot Product9_dotp_13/1
  In2/1 -> mul_Dot Product9_dotp_13/2
  mul_Dot Product9_dotp_13/1 -> mul_Dot Product9_dotp_13_pd1/1
  mul_Dot Product9_dotp_13_pd1/1 -> Out1/1

== system gm_MATE_HDLsolver_myFirstCircuit/ForFPGA/mul_Dot Product9_dotp_14 ==
  In1 : Inport
  In2 : Inport  Port=2
  mul_Dot Product9_dotp_14 : Product  Inputs=**  OutDataTypeStr=single  SampleTime=6.02409638554217e-09
  mul_Dot Product9_dotp_14_pd1 : Delay  DelayLength=6
  Out1 : Outport
  wires:
  In1/1 -> mul_Dot Product9_dotp_14/1
  In2/1 -> mul_Dot Product9_dotp_14/2
  mul_Dot Product9_dotp_14/1 -> mul_Dot Product9_dotp_14_pd1/1
  mul_Dot Product9_dotp_14_pd1/1 -> Out1/1

== system gm_MATE_HDLsolver_myFirstCircuit/ForFPGA/mul_Dot Product9_dotp_15 ==
  In1 : Inport
  In2 : Inport  Port=2
  mul_Dot Product9_dotp_15 : Product  Inputs=**  OutDataTypeStr=single  SampleTime=6.02409638554217e-09
  mul_Dot Product9_dotp_15_pd1 : Delay  DelayLength=6
  Out1 : Outport
  wires:
  In1/1 -> mul_Dot Product9_dotp_15/1
  In2/1 -> mul_Dot Product9_dotp_15/2
  mul_Dot Product9_dotp_15/1 -> mul_Dot Product9_dotp_15_pd1/1
  mul_Dot Product9_dotp_15_pd1/1 -> Out1/1

== system gm_MATE_HDLsolver_myFirstCircuit/ForFPGA/mul_Dot Product9_dotp_2 ==
  In1 : Inport
  In2 : Inport  Port=2
  mul_Dot Product9_dotp_2 : Product  Inputs=**  OutDataTypeStr=single  SampleTime=6.02409638554217e-09
  mul_Dot Product9_dotp_2_pd1 : Delay  DelayLength=6
  Out1 : Outport
  wires:
  In1/1 -> mul_Dot Product9_dotp_2/1
  In2/1 -> mul_Dot Product9_dotp_2/2
  mul_Dot Product9_dotp_2/1 -> mul_Dot Product9_dotp_2_pd1/1
  mul_Dot Product9_dotp_2_pd1/1 -> Out1/1

== system gm_MATE_HDLsolver_myFirstCircuit/ForFPGA/mul_Dot Product9_dotp_3 ==
  In1 : Inport
  In2 : Inport  Port=2
  mul_Dot Product9_dotp_3 : Product  Inputs=**  OutDataTypeStr=single  SampleTime=6.02409638554217e-09
  mul_Dot Product9_dotp_3_pd1 : Delay  DelayLength=6
  Out1 : Outport
  wires:
  In1/1 -> mul_Dot Product9_dotp_3/1
  In2/1 -> mul_Dot Product9_dotp_3/2
  mul_Dot Product9_dotp_3/1 -> mul_Dot Product9_dotp_3_pd1/1
  mul_Dot Product9_dotp_3_pd1/1 -> Out1/1

== system gm_MATE_HDLsolver_myFirstCircuit/ForFPGA/mul_Dot Product9_dotp_4 ==
  In1 : Inport
  In2 : Inport  Port=2
  mul_Dot Product9_dotp_4 : Product  Inputs=**  OutDataTypeStr=single  SampleTime=6.02409638554217e-09
  mul_Dot Product9_dotp_4_pd1 : Delay  DelayLength=6
  Out1 : Outport
  wires:
  In1/1 -> mul_Dot Product9_dotp_4/1
  In2/1 -> mul_Dot Product9_dotp_4/2
  mul_Dot Product9_dotp_4/1 -> mul_Dot Product9_dotp_4_pd1/1
  mul_Dot Product9_dotp_4_pd1/1 -> Out1/1

== system gm_MATE_HDLsolver_myFirstCircuit/ForFPGA/mul_Dot Product9_dotp_5 ==
  In1 : Inport
  In2 : Inport  Port=2
  mul_Dot Product9_dotp_5 : Product  Inputs=**  OutDataTypeStr=single  SampleTime=6.02409638554217e-09
  mul_Dot Product9_dotp_5_pd1 : Delay  DelayLength=6
  Out1 : Outport
  wires:
  In1/1 -> mul_Dot Product9_dotp_5/1
  In2/1 -> mul_Dot Product9_dotp_5/2
  mul_Dot Product9_dotp_5/1 -> mul_Dot Product9_dotp_5_pd1/1
  mul_Dot Product9_dotp_5_pd1/1 -> Out1/1

== system gm_MATE_HDLsolver_myFirstCircuit/ForFPGA/mul_Dot Product9_dotp_6 ==
  In1 : Inport
  In2 : Inport  Port=2
  mul_Dot Product9_dotp_6 : Product  Inputs=**  OutDataTypeStr=single  SampleTime=6.02409638554217e-09
  mul_Dot Product9_dotp_6_pd1 : Delay  DelayLength=6
  Out1 : Outport
  wires:
  In1/1 -> mul_Dot Product9_dotp_6/1
  In2/1 -> mul_Dot Product9_dotp_6/2
  mul_Dot Product9_dotp_6/1 -> mul_Dot Product9_dotp_6_pd1/1
  mul_Dot Product9_dotp_6_pd1/1 -> Out1/1

== system gm_MATE_HDLsolver_myFirstCircuit/ForFPGA/mul_Dot Product9_dotp_7 ==
  In1 : Inport
  In2 : Inport  Port=2
  mul_Dot Product9_dotp_7 : Product  Inputs=**  OutDataTypeStr=single  SampleTime=6.02409638554217e-09
  mul_Dot Product9_dotp_7_pd1 : Delay  DelayLength=6
  Out1 : Outport
  wires:
  In1/1 -> mul_Dot Product9_dotp_7/1
  In2/1 -> mul_Dot Product9_dotp_7/2
  mul_Dot Product9_dotp_7/1 -> mul_Dot Product9_dotp_7_pd1/1
  mul_Dot Product9_dotp_7_pd1/1 -> Out1/1

== system gm_MATE_HDLsolver_myFirstCircuit/ForFPGA/mul_Dot Product9_dotp_8 ==
  In1 : Inport
  In2 : Inport  Port=2
  mul_Dot Product9_dotp_8 : Product  Inputs=**  OutDataTypeStr=single  SampleTime=6.02409638554217e-09
  mul_Dot Product9_dotp_8_pd1 : Delay  DelayLength=6
  Out1 : Outport
  wires:
  In1/1 -> mul_Dot Product9_dotp_8/1
  In2/1 -> mul_Dot Product9_dotp_8/2
  mul_Dot Product9_dotp_8/1 -> mul_Dot Product9_dotp_8_pd1/1
  mul_Dot Product9_dotp_8_pd1/1 -> Out1/1

== system gm_MATE_HDLsolver_myFirstCircuit/ForFPGA/mul_Dot Product9_dotp_9 ==
  In1 : Inport
  In2 : Inport  Port=2
  mul_Dot Product9_dotp_9 : Product  Inputs=**  OutDataTypeStr=single  SampleTime=6.02409638554217e-09
  mul_Dot Product9_dotp_9_pd1 : Delay  DelayLength=6
  Out1 : Outport
  wires:
  In1/1 -> mul_Dot Product9_dotp_9/1
  In2/1 -> mul_Dot Product9_dotp_9/2
  mul_Dot Product9_dotp_9/1 -> mul_Dot Product9_dotp_9_pd1/1
  mul_Dot Product9_dotp_9_pd1/1 -> Out1/1

== system gm_MATE_HDLsolver_myFirstCircuit/ForFPGA/mul_Dot Product_dotp_0 ==
  In1 : Inport
  In2 : Inport  Port=2
  mul_Dot Product_dotp_0 : Product  Inputs=**  OutDataTypeStr=single  SampleTime=6.02409638554217e-09
  mul_Dot Product_dotp_0_pd1 : Delay  DelayLength=6
  Out1 : Outport
  wires:
  In1/1 -> mul_Dot Product_dotp_0/1
  In2/1 -> mul_Dot Product_dotp_0/2
  mul_Dot Product_dotp_0/1 -> mul_Dot Product_dotp_0_pd1/1
  mul_Dot Product_dotp_0_pd1/1 -> Out1/1

== system gm_MATE_HDLsolver_myFirstCircuit/ForFPGA/mul_Dot Product_dotp_1 ==
  In1 : Inport
  In2 : Inport  Port=2
  mul_Dot Product_dotp_1 : Product  Inputs=**  OutDataTypeStr=single  SampleTime=6.02409638554217e-09
  mul_Dot Product_dotp_1_pd1 : Delay  DelayLength=6
  Out1 : Outport
  wires:
  In1/1 -> mul_Dot Product_dotp_1/1
  In2/1 -> mul_Dot Product_dotp_1/2
  mul_Dot Product_dotp_1/1 -> mul_Dot Product_dotp_1_pd1/1
  mul_Dot Product_dotp_1_pd1/1 -> Out1/1

== system gm_MATE_HDLsolver_myFirstCircuit/ForFPGA/mul_Dot Product_dotp_10 ==
  In1 : Inport
  In2 : Inport  Port=2
  mul_Dot Product_dotp_10 : Product  Inputs=**  OutDataTypeStr=single  SampleTime=6.02409638554217e-09
  mul_Dot Product_dotp_10_pd1 : Delay  DelayLength=6
  Out1 : Outport
  wires:
  In1/1 -> mul_Dot Product_dotp_10/1
  In2/1 -> mul_Dot Product_dotp_10/2
  mul_Dot Product_dotp_10/1 -> mul_Dot Product_dotp_10_pd1/1
  mul_Dot Product_dotp_10_pd1/1 -> Out1/1

== system gm_MATE_HDLsolver_myFirstCircuit/ForFPGA/mul_Dot Product_dotp_11 ==
  In1 : Inport
  In2 : Inport  Port=2
  mul_Dot Product_dotp_11 : Product  Inputs=**  OutDataTypeStr=single  SampleTime=6.02409638554217e-09
  mul_Dot Product_dotp_11_pd1 : Delay  DelayLength=6
  Out1 : Outport
  wires:
  In1/1 -> mul_Dot Product_dotp_11/1
  In2/1 -> mul_Dot Product_dotp_11/2
  mul_Dot Product_dotp_11/1 -> mul_Dot Product_dotp_11_pd1/1
  mul_Dot Product_dotp_11_pd1/1 -> Out1/1

== system gm_MATE_HDLsolver_myFirstCircuit/ForFPGA/mul_Dot Product_dotp_12 ==
  In1 : Inport
  In2 : Inport  Port=2
  mul_Dot Product_dotp_12 : Product  Inputs=**  OutDataTypeStr=single  SampleTime=6.02409638554217e-09
  mul_Dot Product_dotp_12_pd1 : Delay  DelayLength=6
  Out1 : Outport
  wires:
  In1/1 -> mul_Dot Product_dotp_12/1
  In2/1 -> mul_Dot Product_dotp_12/2
  mul_Dot Product_dotp_12/1 -> mul_Dot Product_dotp_12_pd1/1
  mul_Dot Product_dotp_12_pd1/1 -> Out1/1

== system gm_MATE_HDLsolver_myFirstCircuit/ForFPGA/mul_Dot Product_dotp_13 ==
  In1 : Inport
  In2 : Inport  Port=2
  mul_Dot Product_dotp_13 : Product  Inputs=**  OutDataTypeStr=single  SampleTime=6.02409638554217e-09
  mul_Dot Product_dotp_13_pd1 : Delay  DelayLength=6
  Out1 : Outport
  wires:
  In1/1 -> mul_Dot Product_dotp_13/1
  In2/1 -> mul_Dot Product_dotp_13/2
  mul_Dot Product_dotp_13/1 -> mul_Dot Product_dotp_13_pd1/1
  mul_Dot Product_dotp_13_pd1/1 -> Out1/1

== system gm_MATE_HDLsolver_myFirstCircuit/ForFPGA/mul_Dot Product_dotp_14 ==
  In1 : Inport
  In2 : Inport  Port=2
  mul_Dot Product_dotp_14 : Product  Inputs=**  OutDataTypeStr=single  SampleTime=6.02409638554217e-09
  mul_Dot Product_dotp_14_pd1 : Delay  DelayLength=6
  Out1 : Outport
  wires:
  In1/1 -> mul_Dot Product_dotp_14/1
  In2/1 -> mul_Dot Product_dotp_14/2
  mul_Dot Product_dotp_14/1 -> mul_Dot Product_dotp_14_pd1/1
  mul_Dot Product_dotp_14_pd1/1 -> Out1/1

== system gm_MATE_HDLsolver_myFirstCircuit/ForFPGA/mul_Dot Product_dotp_15 ==
  In1 : Inport
  In2 : Inport  Port=2
  mul_Dot Product_dotp_15 : Product  Inputs=**  OutDataTypeStr=single  SampleTime=6.02409638554217e-09
  mul_Dot Product_dotp_15_pd1 : Delay  DelayLength=6
  Out1 : Outport
  wires:
  In1/1 -> mul_Dot Product_dotp_15/1
  In2/1 -> mul_Dot Product_dotp_15/2
  mul_Dot Product_dotp_15/1 -> mul_Dot Product_dotp_15_pd1/1
  mul_Dot Product_dotp_15_pd1/1 -> Out1/1

== system gm_MATE_HDLsolver_myFirstCircuit/ForFPGA/mul_Dot Product_dotp_2 ==
  In1 : Inport
  In2 : Inport  Port=2
  mul_Dot Product_dotp_2 : Product  Inputs=**  OutDataTypeStr=single  SampleTime=6.02409638554217e-09
  mul_Dot Product_dotp_2_pd1 : Delay  DelayLength=6
  Out1 : Outport
  wires:
  In1/1 -> mul_Dot Product_dotp_2/1
  In2/1 -> mul_Dot Product_dotp_2/2
  mul_Dot Product_dotp_2/1 -> mul_Dot Product_dotp_2_pd1/1
  mul_Dot Product_dotp_2_pd1/1 -> Out1/1

== system gm_MATE_HDLsolver_myFirstCircuit/ForFPGA/mul_Dot Product_dotp_3 ==
  In1 : Inport
  In2 : Inport  Port=2
  mul_Dot Product_dotp_3 : Product  Inputs=**  OutDataTypeStr=single  SampleTime=6.02409638554217e-09
  mul_Dot Product_dotp_3_pd1 : Delay  DelayLength=6
  Out1 : Outport
  wires:
  In1/1 -> mul_Dot Product_dotp_3/1
  In2/1 -> mul_Dot Product_dotp_3/2
  mul_Dot Product_dotp_3/1 -> mul_Dot Product_dotp_3_pd1/1
  mul_Dot Product_dotp_3_pd1/1 -> Out1/1

== system gm_MATE_HDLsolver_myFirstCircuit/ForFPGA/mul_Dot Product_dotp_4 ==
  In1 : Inport
  In2 : Inport  Port=2
  mul_Dot Product_dotp_4 : Product  Inputs=**  OutDataTypeStr=single  SampleTime=6.02409638554217e-09
  mul_Dot Product_dotp_4_pd1 : Delay  DelayLength=6
  Out1 : Outport
  wires:
  In1/1 -> mul_Dot Product_dotp_4/1
  In2/1 -> mul_Dot Product_dotp_4/2
  mul_Dot Product_dotp_4/1 -> mul_Dot Product_dotp_4_pd1/1
  mul_Dot Product_dotp_4_pd1/1 -> Out1/1

== system gm_MATE_HDLsolver_myFirstCircuit/ForFPGA/mul_Dot Product_dotp_5 ==
  In1 : Inport
  In2 : Inport  Port=2
  mul_Dot Product_dotp_5 : Product  Inputs=**  OutDataTypeStr=single  SampleTime=6.02409638554217e-09
  mul_Dot Product_dotp_5_pd1 : Delay  DelayLength=6
  Out1 : Outport
  wires:
  In1/1 -> mul_Dot Product_dotp_5/1
  In2/1 -> mul_Dot Product_dotp_5/2
  mul_Dot Product_dotp_5/1 -> mul_Dot Product_dotp_5_pd1/1
  mul_Dot Product_dotp_5_pd1/1 -> Out1/1

== system gm_MATE_HDLsolver_myFirstCircuit/ForFPGA/mul_Dot Product_dotp_6 ==
  In1 : Inport
  In2 : Inport  Port=2
  mul_Dot Product_dotp_6 : Product  Inputs=**  OutDataTypeStr=single  SampleTime=6.02409638554217e-09
  mul_Dot Product_dotp_6_pd1 : Delay  DelayLength=6
  Out1 : Outport
  wires:
  In1/1 -> mul_Dot Product_dotp_6/1
  In2/1 -> mul_Dot Product_dotp_6/2
  mul_Dot Product_dotp_6/1 -> mul_Dot Product_dotp_6_pd1/1
  mul_Dot Product_dotp_6_pd1/1 -> Out1/1

== system gm_MATE_HDLsolver_myFirstCircuit/ForFPGA/mul_Dot Product_dotp_7 ==
  In1 : Inport
  In2 : Inport  Port=2
  mul_Dot Product_dotp_7 : Product  Inputs=**  OutDataTypeStr=single  SampleTime=6.02409638554217e-09
  mul_Dot Product_dotp_7_pd1 : Delay  DelayLength=6
  Out1 : Outport
  wires:
  In1/1 -> mul_Dot Product_dotp_7/1
  In2/1 -> mul_Dot Product_dotp_7/2
  mul_Dot Product_dotp_7/1 -> mul_Dot Product_dotp_7_pd1/1
  mul_Dot Product_dotp_7_pd1/1 -> Out1/1

== system gm_MATE_HDLsolver_myFirstCircuit/ForFPGA/mul_Dot Product_dotp_8 ==
  In1 : Inport
  In2 : Inport  Port=2
  mul_Dot Product_dotp_8 : Product  Inputs=**  OutDataTypeStr=single  SampleTime=6.02409638554217e-09
  mul_Dot Product_dotp_8_pd1 : Delay  DelayLength=6
  Out1 : Outport
  wires:
  In1/1 -> mul_Dot Product_dotp_8/1
  In2/1 -> mul_Dot Product_dotp_8/2
  mul_Dot Product_dotp_8/1 -> mul_Dot Product_dotp_8_pd1/1
  mul_Dot Product_dotp_8_pd1/1 -> Out1/1

== system gm_MATE_HDLsolver_myFirstCircuit/ForFPGA/mul_Dot Product_dotp_9 ==
  In1 : Inport
  In2 : Inport  Port=2
  mul_Dot Product_dotp_9 : Product  Inputs=**  OutDataTypeStr=single  SampleTime=6.02409638554217e-09
  mul_Dot Product_dotp_9_pd1 : Delay  DelayLength=6
  Out1 : Outport
  wires:
  In1/1 -> mul_Dot Product_dotp_9/1
  In2/1 -> mul_Dot Product_dotp_9/2
  mul_Dot Product_dotp_9/1 -> mul_Dot Product_dotp_9_pd1/1
  mul_Dot Product_dotp_9_pd1/1 -> Out1/1

== system gm_MATE_HDLsolver_myFirstCircuit/MATEBUCK/Input current ==
  CS_input : fl_lib/Electrical/Electrical Sensors/Current Sensor
  PS-Simulink Converter1 : nesl_utility/PS-Simulink Converter  PhysicalDomain=network_engine_domain  SubClassName=ps_output  LeftPortType=input  RightPortType=output  PseudoPeriodic=off  Frequencies=[]  VectorFormat=inherit  Unit=inherit  AffineConversion=off
  + : PMIOPort  Side=Left
  - : PMIOPort  Port=2  Side=Right
  i : Outport
  wires:
  PS-Simulink Converter1/1 -> i/1
  connections:
  CS_input/RConn2 -- -/RConn1
  CS_input/LConn1 -- +/RConn1
  PS-Simulink Converter1/LConn1 -- CS_input/RConn1

== system gm_MATE_HDLsolver_myFirstCircuit/MATEBUCK/Load current ==
  CSLoad : fl_lib/Electrical/Electrical Sensors/Current Sensor
  PS-Simulink Converter1 : nesl_utility/PS-Simulink Converter  PhysicalDomain=network_engine_domain  SubClassName=ps_output  LeftPortType=input  RightPortType=output  PseudoPeriodic=off  Frequencies=[]  VectorFormat=inherit  Unit=inherit  AffineConversion=off
  + : PMIOPort  Side=Left
  - : PMIOPort  Port=2  Side=Right
  i : Outport
  wires:
  PS-Simulink Converter1/1 -> i/1
  connections:
  PS-Simulink Converter1/LConn1 -- CSLoad/RConn1
  CSLoad/LConn1 -- +/RConn1
  CSLoad/RConn2 -- -/RConn1

== system gm_MATE_HDLsolver_myFirstCircuit/MATEBUCK/current measure1 ==
  Current Sensor2 : fl_lib/Electrical/Electrical Sensors/Current Sensor
  PS-Simulink Converter1 : nesl_utility/PS-Simulink Converter  PhysicalDomain=network_engine_domain  SubClassName=ps_output  LeftPortType=input  RightPortType=output  PseudoPeriodic=off  Frequencies=[]  VectorFormat=inherit  Unit=inherit  AffineConversion=off
  + : PMIOPort  Side=Left
  - : PMIOPort  Port=2  Side=Right
  i : Outport
  wires:
  PS-Simulink Converter1/1 -> i/1
  connections:
  PS-Simulink Converter1/LConn1 -- Current Sensor2/RConn1
  Current Sensor2/LConn1 -- +/RConn1
  Current Sensor2/RConn2 -- -/RConn1

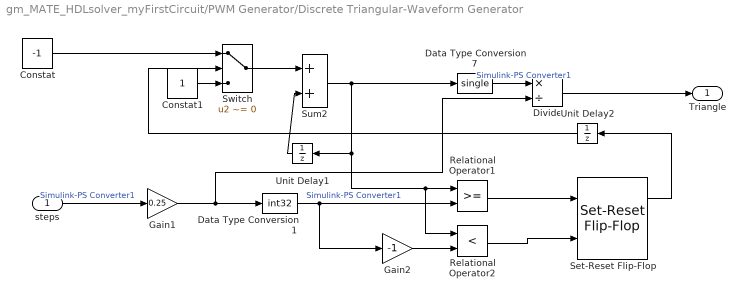
== system gm_MATE_HDLsolver_myFirstCircuit/PWM Generator/Discrete Triangular-Waveform Generator ==
  steps : Inport
  Constat : Constant  Value=-1  OutDataTypeStr=int32
  Constat1 : Constant  OutDataTypeStr=int32
  Data Type Conversion1 : DataTypeConversion  OutDataTypeStr=int32  RndMeth=Nearest  SaturateOnIntegerOverflow=off
  Data Type Conversion7 : DataTypeConversion  OutDataTypeStr=single  RndMeth=Nearest  SaturateOnIntegerOverflow=off
  Divide : Product  Inputs=*/
  Gain1 : Gain  Gain=0.25  SaturateOnIntegerOverflow=on  OutDataTypeStr=Inherit: Same as input  ParamDataTypeStr=Inherit: Same as input
  Gain2 : Gain  Gain=-1  SaturateOnIntegerOverflow=on  OutDataTypeStr=Inherit: Same as input  ParamDataTypeStr=Inherit: Same as input
  Relational Operator1 : RelationalOperator
  Relational Operator2 : RelationalOperator  Operator=<
  Set-Reset Flip-Flop : eeGeneralControl/Set-Reset Flip-Flop  LabelModeActiveChoice=Discrete  UndefState=Set  Q0=0  Ts=Ts
      settings: LibrarySourceBlock=ee_sl_lib/General Control/Set-Reset Flip-Flop
  Sum2 : Sum  InputSameDT=on  SaturateOnIntegerOverflow=on  OutDataTypeStr=Inherit: Same as first input
  Switch : Switch  Criteria=u2 ~= 0
  Unit Delay1 : UnitDelay  SampleTime=Ts  HasFrameUpgradeWarning=on
  Unit Delay2 : UnitDelay  SampleTime=Ts  HasFrameUpgradeWarning=on
  Triangle : Outport  InitialOutput=0  VectorParamsAs1DForOutWhenUnconnected=off
  wires:
  Data Type Conversion1/1 -> Relational Operator1/2, Gain2/1  "Simulink-PS Converter1"
  steps/1 -> Gain1/1  "Simulink-PS Converter1"
  Data Type Conversion7/1 -> Divide/1  "Simulink-PS Converter1"
  Divide/1 -> Triangle/1
  Unit Delay2/1 -> Switch/2
  Set-Reset Flip-Flop/1 -> Unit Delay2/1
  Relational Operator2/1 -> Set-Reset Flip-Flop/2
  Gain2/1 -> Relational Operator2/2
  Relational Operator1/1 -> Set-Reset Flip-Flop/1
  Gain1/1 -> Data Type Conversion1/1, Divide/2
  Sum2/1 -> Data Type Conversion7/1, Unit Delay1/1, Relational Operator1/1, Relational Operator2/1
  Unit Delay1/1 -> Sum2/2
  Switch/1 -> Sum2/1
  Constat1/1 -> Switch/3
  Constat/1 -> Switch/1
